simulink model "G"  (R2021a)
settings: Solver=VariableStepAuto  StartTime=0.0  StopTime=10.0  RelTol=1e-3
libraries: simulink x1
settings Model: Creator=lmeissne  LastModifiedBy=lmeissne

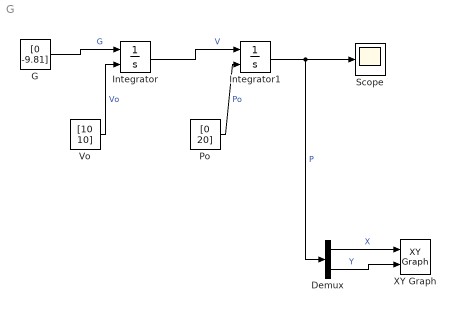
== system G ==
  Demux : Demux  Outputs=2
  G : Constant  Value=[0 -9.81]
  Integrator : Integrator  InitialConditionSource=external
  Integrator1 : Integrator  InitialConditionSource=external
  Po : Constant  Value=[0 20]
  Scope : Scope
  Vo : Constant  Value=[10 10]
  XY Graph : simulink/Sinks/XY Graph  xmin=0  xmax=100  ymin=-400  ymax=50  st=-1
  wires:
  G/1 -> Integrator/1  "G"
  Integrator/1 -> Integrator1/1  "V"
  Vo/1 -> Integrator/2  "Vo"
  Po/1 -> Integrator1/2  "Po"
  Integrator1/1 -> Demux/1, Scope/1  "P"
  Demux/1 -> XY Graph/1  "X"
  Demux/2 -> XY Graph/2  "Y"
